simulink model "helicopter_ver19g"  (R2025b)
settings: Solver=ode3  StartTime=0.0  StopTime=120  FixedStep=0.01  RelTol=1e-9  EnableMultiTasking=on
InitFcn:
  | % Plant parameters
  | T=0.1;
  | gi=0.0375;
  | k=0.103825;
  | wn=1.27;
  | 
  | % Controller
  | numG = 3;
  | denG = 1;
  | numF = 1;
  | denF = 1;
values from neighbouring files (symbols this model uses):
  Kd = 80.0    (= 80)    [run_optimization.m]
  Ki = 0.001    [run_optimization.m]
  Kp = 150.0    (= 150)    [run_optimization.m]
  N = 200    [run_optimization.m]
libraries: simulink x2, slpidlib x1
settings Model: Creator=mgsanz  LastModifiedBy=aloti
settings SolverCC: AlgebraicLoopSolver=TrustRegion
settings DataIOCC: LimitDataPoints=on  SaveFormat=Array  SignalLoggingSaveFormat=ModelDataLogs  ReturnWorkspaceOutputs=off
settings OptimizationCC: ExpressionDepthLimit=2147483647.0  InitFltsAndDblsToZero=on  LifeSpan=inf
settings DebuggingCC: SaveWithParameterizedLinksMsg=none  UnderspecifiedInitializationDetection=Classic  MergeDetectMultiDrivingBlocksExec=none  SignalResolutionControl=TryResolveAllWithWarning  SolverPrmCheckMsg=warning  MultiTaskDSMMsg=warning  MultiTaskCondExecSysMsg=none  FcnCallInpInsideContextMsg=warning  UnconnectedInputMsg=warning  UnconnectedOutputMsg=warning  UnconnectedLineMsg=warning  StateNameClashWarn=warning  SFUnexpectedBacktrackingDiag=warning  SFNoUnconditionalDefaultTransitionDiag=warning  SFExecutionAtInitializationDiag=none  ArithmeticOperatorsInVariantConditions=warning
settings HardwareCC: ProdBitPerPointer=32.0  ProdBitPerSizeT=32.0  ProdBitPerPtrDiffT=32.0  ProdLargestAtomicFloat=None  ProdIntDivRoundTo=Undefined  ProdEndianess=Unspecified  ProdWordSize=32.0  ProdHWDeviceType=32-bit Generic
settings ModelReferenceCC: PropagateSignalLabelsOutOfModel=off
settings SFSimCC: SimUseLocalCustomCode=off  CustomCodeUndefinedFunction=UseInterfaceOnly
settings RTWCC: RTWUseLocalCustomCode=off  GPUComputeCapability=3.5
settings CodeAppCC: StateflowObjectComments=on
settings GRTTargetCC: TargetFcnLib=ansi_tfl_tmw.mat  TargetLangStandard=C89/C90 (ANSI)  CombineOutputUpdateFcns=off  GRTInterface=on
settings ConfigComp: CovMetricSettings=dw  CovSaveCumulativeToWorkspaceVar=on  CovSaveSingleToWorkspaceVar=on  CovExternalEMLEnable=off  CovSFcnEnable=off

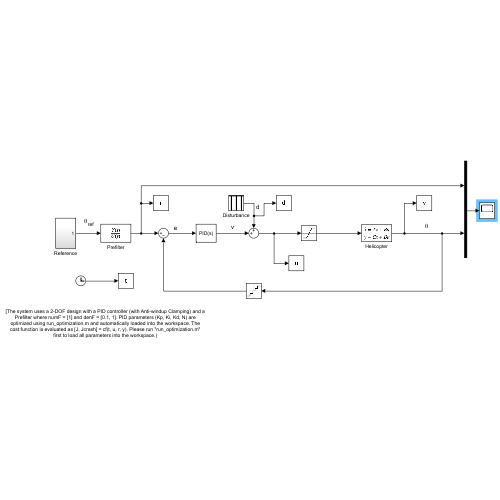
[thumbnail: Simulink's stored preview of the top-level diagram]
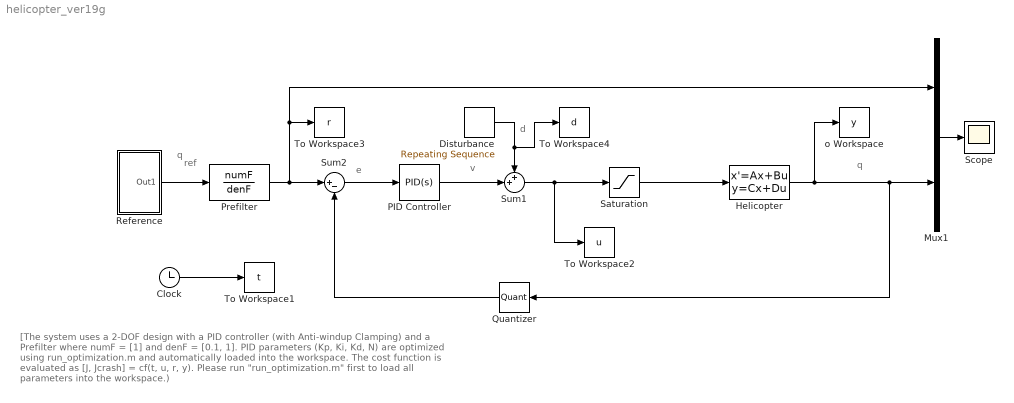
== system helicopter_ver19g ==
  note: q
  note: q
  note: ref
  note: v
  note: e
  note: d
  note: [The system uses a 2-DOF design with a PID controller (with Anti-windup Clamping) and a Prefilter where numF = [1] and denF = [0.1, 1]. PID parameters (Kp, Ki, Kd, N) are optimized using run_optimization.m and automatically loaded into the workspace. The cost function is evaluated as [J, Jcrash] = cf(t, u, r, y). Please run "run_optimization.m" first to load all parameters into the workspace.)
  Clock : Clock
  Disturbance : simulink/Sources/Repeating Sequence  rep_seq_t="[0 65 65.01 67 67.01  120]"  rep_seq_y="[0  0  -17 -17   0        0]"
  Helicopter : StateSpace  A=[0 1; -wn^2 -2*gi*wn]  B=[0; k*wn^2]  C=[1 0]  D=0  InitialCondition=[-20*pi/180; 0]
  Mux1 : Mux  Inputs=2
  PID Controller : slpidlib/PID Controller  Controller=PID  Form=Parallel  TimeDomain=Continuous-time  UseExternalTs=off  SampleTime=-1  IntegratorMethod=Forward Euler  FilterMethod=Forward Euler  ControllerParametersSource=internal  P=Kp  I=Ki  UseKiTs=on  D=Kd  UseExternalDerivativeSource=off  N=N  UseFilter=on  TunerSelectOption=Transfer Function Based (PID Tuner App)  InitialConditionSource=internal  InitialConditionForIntegrator=0  InitialConditionForFilter=0  DifferentiatorICPrevScaledInput=0  ExternalReset=none  TrackingMode=off  Kt=1  LimitOutput=off  SatLimitsSource=internal  UpperSaturationLimit=inf  LowerSaturationLimit=-inf  LinearizeAsGain=on  AntiWindupMode=none  Kb=1  LimitIntegrator=off  UpperIntegratorSaturationLimit=inf  LowerIntegratorSaturationLimit=-inf  POutMin=[]  POutMax=[]  IOutMin=[]  IOutMax=[]  DOutMin=[]  DOutMax=[]  NOutMin=[]  NOutMax=[]  SumOutMin=[]  SumOutMax=[]  SaturationOutMin=[]  SaturationOutMax=[]  PParamMin=[]  PParamMax=[]  IParamMin=[]  IParamMax=[]  DParamMin=[]  DParamMax=[]  NParamMin=[]  NParamMax=[]  KbParamMin=[]  KbParamMax=[]  KtParamMin=[]  KtParamMax=[]  KbOutMin=[]  KbOutMax=[]  KtOutMin=[]  KtOutMax=[]  IntegratorOutMin=[]  IntegratorOutMax=[]  FilterOutMin=[]  FilterOutMax=[]  SumI1OutMin=[]  SumI1OutMax=[]  SumI2OutMin=[]  SumI2OutMax=[]  SumI3OutMin=[]  SumI3OutMax=[]  SumI4OutMin=[]  SumI4OutMax=[]  SumDOutMin=[]  SumDOutMax=[]  DifferentiatorOutMin=[]  DifferentiatorOutMax=[]  FilterDiffOutCoefMin=[]  FilterDiffOutCoefMax=[]  ReciprocalOutMin=[]  ReciprocalOutMax=[]  SumDenOutMin=[]  SumDenOutMax=[]  SumNumOutMin=[]  SumNumOutMax=[]  DivideOutMin=[]  DivideOutMax=[]  UdiffTsProdOutMin=[]  UdiffTsProdOutMax=[]  NTsProdOutMin=[]  NTsProdOutMax=[]  UintegralTsProdOutMin=[]  UintegralTsProdOutMax=[]  UngainTsProdOutMin=[]  UngainTsProdOutMax=[]  ClampingZeroOutDataTypeStr=Inherit: Inherit via back propagation  ClampingZeroOutMin=[]  ClampingZeroOutMax=[]  FilterDenConstantOutDataTypeStr=Inherit: Inherit via back propagation  FilterDenConstantOutMin=[]  FilterDenConstantOutMax=[]  PCopyOutDataTypeStr=Inherit: Inherit via back propagation  PCopyOutMin=[]  PCopyOutMax=[]  NCopyOutDataTypeStr=Inherit: Inherit via back propagation  NCopyOutMin=[]  NCopyOutMax=[]  IntegratorContinuousStateAttributes=''  IntegratorStateMustResolveToSignalObject=off  IntegratorRTWStateStorageClass=Auto  FilterContinuousStateAttributes=''  FilterStateMustResolveToSignalObject=off  FilterRTWStateStorageClass=Auto  ParallelPVariant=InternalParameters  IdealPVariant=Disabled  IVariant=InternalParameters  DVariant=InternalParameters  IntegratorVariant=Continuous  SatVariant=Disabled  AWVariant=Passthrough  PCopyVariant=Disabled  TRVariant=Disabled  FdbkBlocksVariant=Forward  IdealPFdbkVariant=Disabled  SatFdbkVariant=Disabled  DerivativeFilterVariant=ContFilter  NVariant=InternalParameters  NCopyVariant=Disabled  FilterICVariant=InternalICsFilter  IntegratorICVariant=InternalICs  ExternalResetVariant=Disabled  TRSumVariant=Passthrough  SumFdbkVariant=Disabled  SumVariant=Sum_PID  TsampFilterVariant=InternalTs  TsampNgainVariant=Passthrough  TsampIntegralVariant=Disabled_SignalSpec  ExternalSaturationOutDataTypeStr=Inherit: Same as second input  DerivativeSourceVariant=ErrorSignal  PreIntVariant=InternalPreInt
  Prefilter : TransferFcn  Numerator=numF  Denominator=denF
  Quantizer : Quantizer  QuantizationInterval=0.0015
  Reference : Subsystem
  Saturation : Saturate  UpperLimit=2.6  LowerLimit=-17.4
  Scope : Scope
      settings: TimeSpan=120  ActiveDisplayYMinimum=-2.5343821096125274  ActiveDisplayYMaximum=2.1607843292857827
  Sum1 : Sum  Inputs=++|
  Sum2 : Sum  Inputs=|+-
  To Workspace1 : ToWorkspace  VariableName=t  SampleTime=-1
  To Workspace2 : ToWorkspace  VariableName=u  SampleTime=-1
  To Workspace3 : ToWorkspace  VariableName=r  SampleTime=-1
  To Workspace4 : ToWorkspace  VariableName=d  SampleTime=-1
  o Workspace : ToWorkspace  VariableName=y  SampleTime=-1
  wires:
  Sum1/1 -> To Workspace2/1, Saturation/1
  Sum2/1 -> PID Controller/1
  Mux1/1 -> Scope/1
  Reference/1(Out1) -> Prefilter/1
  Clock/1 -> To Workspace1/1
  Disturbance/1 -> Sum1/1, To Workspace4/1
  PID Controller/1 -> Sum1/2
  Helicopter/1 -> Mux1/2, Quantizer/1, o Workspace/1
  Quantizer/1 -> Sum2/2
  Saturation/1 -> Helicopter/1
  Prefilter/1 -> Sum2/1, Mux1/1, To Workspace3/1

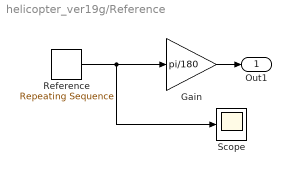
== system helicopter_ver19g/Reference ==
  Gain : Gain  Gain=pi/180
  Reference : simulink/Sources/Repeating Sequence  rep_seq_t="[0      30    50    80    80.01    95    97    99   101   103   105   109    113   115   120]"  rep_seq_y="[-20  -20   0   0   10  10  4.3 -0.8 -5.3 -9.2 -12.5 -17.3 -19.7     -20       -20]"
  Scope : Scope
      settings: TimeSpan=120  ActiveDisplayYMinimum=-23.75  ActiveDisplayYMaximum=13.75
  Out1 : Outport
  wires:
  Reference/1 -> Gain/1, Scope/1
  Gain/1 -> Out1/1
